simulink model "myrocket"  (R2014b)
settings: Solver=ode45  StartTime=0.0  StopTime=10.0  RelTol=1e-3
settings Model: Creator=sigurd  LastModifiedBy=sigurd

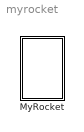
== system myrocket ==
  MyRocket : Subsystem

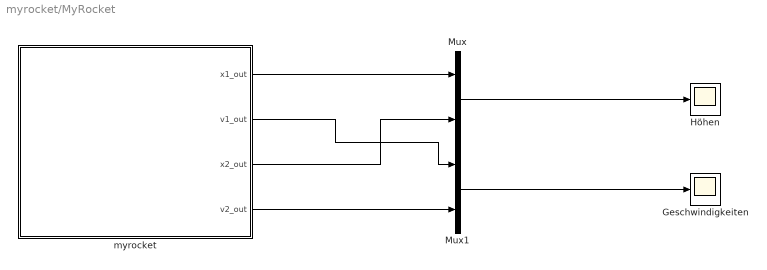
== system myrocket/MyRocket ==
  Geschwindigkeiten : Scope
  Höhen : Scope
  Mux : Mux  Inputs=2
  Mux1 : Mux  Inputs=2
  myrocket : Stateflow chart  TreatAsAtomicUnit=on  mask{m1_leer=500, m2_leer=1000, St1_Treibstoff=4000, St2_Treibstoff=1500, Durchsatz_1=20, Durchsatz_2=15, SchubProDurchsatz=4000}
      mask prompts: m1_leer "m1_leer [kg]"; m2_leer "m2_leer [kg]"; St1_Treibstoff "m1_Treibstoff [kg]"; St2_Treibstoff "m2_Treibstoff [kg]"; Durchsatz_1 "Durchsatz 1 [kg/s]"; Durchsatz_2 "Durchsatz 2 [kg/s]"; SchubProDurchsatz "SchubProDurchsatz [N/(kg/s)]"
  wires:
  myrocket/4(v2_out) -> Mux1/2
  myrocket/1(x1_out) -> Mux/1
  myrocket/3(x2_out) -> Mux/2
  Mux1/1 -> Geschwindigkeiten/1
  Mux/1 -> Höhen/1
  myrocket/2(v1_out) -> Mux1/1

== stateflow chart myrocket/MyRocket/myrocket ==
  settings: updateMethod=CONTINUOUS
  state Antriebslos
    du:
    % Derivatives
    [v1_dot, v2_dot] = Acc3();
    x1_dot=v1;x2_dot = v2;
    m1_dot=0;
    m2_dot=0;
    % Output
    x1_out=x1;x2_out=x2;
    v1_out=v1;v2_out=v2;
  state Stufe2
    du:
    % Derivatives
    [v1_dot, v2_dot] = Acc2();
    x1_dot=v1;x2_dot = v2;
    m1_dot=0;
    m2_dot= - Durchsatz_2;
    % Output
    x1_out=x1;x2_out=x2;
    v1_out=v1;v2_out=v2;
  state Stufe1
    du:
    % Derivatives
    [v1_dot, v2_dot] = Acc1();
    x1_dot=v1;x2_dot = v2;
    m1_dot = - Durchsatz_1;
    m2_dot=0;
    % Output
    x1_out=x1;x2_out=x2;
    v1_out=v1;v2_out=v2;
  Stufe2 -> Antriebslos : [m2 <= m2_leer]
  (default) -> Stufe1 : {init()}
  Stufe1 -> Stufe2 : [m1 <= m1_leer]
  data: a1 function_output; a2 function_output; a1 function_output; a2 function_output; a1 function_output; a2 function_output; x1_out output; v1_out output; x2_out output; v2_out output; x1 local; x2 local; v1 local; v2 local; rE constant double =6378*1000; mE constant double =5.9736*10^24; G constant double =66.743*10^(-12); m1_leer parameter; m2_leer parameter; St1_Treibstoff parameter; St2_Treibstoff parameter; Durchsatz_1 parameter; Durchsatz_2 parameter; SchubProDurchsatz parameter; m1 local; m2 local
  data x1 settings: updateMethod=SF_CONTINUOUS_TIME_DATA
  data x2 settings: updateMethod=SF_CONTINUOUS_TIME_DATA
  data v1 settings: updateMethod=SF_CONTINUOUS_TIME_DATA
  data v2 settings: updateMethod=SF_CONTINUOUS_TIME_DATA
  data m1 settings: updateMethod=SF_CONTINUOUS_TIME_DATA
  data m2 settings: updateMethod=SF_CONTINUOUS_TIME_DATA
  function [a1,a2] = Acc3:
    | function [a1,a2] = Acc3
    |  
    | r1 = x1 + rE;
    | Fs1 = G * (mE * m1) / (r1*r1);
    | r2 = x2 + rE;
    | Fs2 = G * (mE * m2) / (r2*r2);
    | 
    | a1 = - Fs1 / m1;
    | a2 = - Fs2 / m2;
  function init:
    | function init
    |  
    | x1 = 0;
    | v1 = 0;
    | 
    | x2 = 0;
    | v2 = 0;
    | 
    | m1 = m1_leer + St1_Treibstoff;
    | m2 = m2_leer + St2_Treibstoff;
  function [a1,a2] = Acc2:
    | function [a1,a2] = Acc2
    |  
    | r1 = x1 + rE;
    | Fs1 = G * (mE * m1) / (r1*r1);
    | r2 = x2 + rE;
    | Fs2 = G * (mE * m2) / (r2*r2);
    | Schubkraft_2 = Durchsatz_2 * SchubProDurchsatz;
    | 
    | a1 = - Fs1 / m1;
    | a2 = (Schubkraft_2- Fs2) / m2;
  function [a1,a2] = Acc1:
    | function [a1,a2] = Acc1
    | 
    | mR = m1 + m2;
    | r1 = x1 + rE;
    | Fs1 = G * (mE * mR) / (r1*r1);
    | Schubkraft_1 = Durchsatz_1 * SchubProDurchsatz;
    | 
    | a = (Schubkraft_1 - Fs1) / (m1+m2);
    | a1 = a;
    | a2 = a;
